simulink subsystem "PvtSubSys_LSM"  (R2020b)
settings: Solver=VariableStepAuto  StartTime=0.0  StopTime=10.0  RelTol=1e-3
values from neighbouring files (symbols this model uses):
  P_LSM_ALC_Enable = 0.0    [LSM_Parameter.sldd]
  P_LSM_DOP_C0_EN_Limit = 0.8    [LSM_Parameter.sldd]
  P_LSM_DOP_C0_out_Limit = 2.0    [LSM_Parameter.sldd]
  P_LSM_DOP_C1_EN_Limit : value not decoded    [LSM_Parameter.sldd]
  P_LSM_DOP_C1_out_Limit : value not decoded    [LSM_Parameter.sldd]
  P_LSM_DOP_C1AndC2_Lim_X : value not decoded    [LSM_Parameter.sldd]
  P_LSM_DOP_C2_EN_Limit : value not decoded    [LSM_Parameter.sldd]
  P_LSM_DOP_C2_out_Limit : value not decoded    [LSM_Parameter.sldd]
  P_LSM_DOP_In_Pre2Dop_Dis = 1.0    [LSM_Parameter.sldd]
  P_LSM_DOP_Out_Pre2Dop_Dis = 2.0    [LSM_Parameter.sldd]
  P_LSM_DOP_PreDis_X : value not decoded    [LSM_Parameter.sldd]
  P_LSM_DOP_PreDis_Y : value not decoded    [LSM_Parameter.sldd]
  P_LSM_DOPValid_CheckTime = 0.06    [LSM_Parameter.sldd]
  P_LSM_DoubleLine_Curr2Cent_Dislimit = 0.5    [LSM_Parameter.sldd]
  P_LSM_DoubleLine_Dop2Cent_Dislimit = 0.5    [LSM_Parameter.sldd]
  P_LSM_DoubleLine_DOPOut_C1 : value not decoded    [LSM_Parameter.sldd]
  P_LSM_DoubleLine_Pre2Cent_Dislimit = 1.0    [LSM_Parameter.sldd]
  P_LSM_IFV2CenterAxis = 0.0    [LSM_Parameter.sldd]
  P_LSM_IFV2RearAxis = 0.0    [LSM_Parameter.sldd]
  P_LSM_LineSTD_Limit = 0.15    [LSM_Parameter.sldd]
  P_LSM_NOH_Switch = 0.0    [LSM_Parameter.sldd]
  P_LSM_Pre_t = 0.0    [LSM_Parameter.sldd]
  P_LSM_SingleLine_Cent2Edge_Dislimit = 100.0    [LSM_Parameter.sldd]
  P_LSM_SingleLine_Curr2Cent_Dislimit = 0.2    [LSM_Parameter.sldd]
  P_LSM_SingleLine_Dop2Cent_Dislimit = 0.2    [LSM_Parameter.sldd]
  P_LSM_SingleLine_DOPOut_C1 : value not decoded    [LSM_Parameter.sldd]
  P_LSM_SingleLine_Pre2Cent_Dislimit = 0.5    [LSM_Parameter.sldd]
undefined symbols (not defined in the file or in its folder): P_LSM_LineWijCal_C12, P_LSM_LineWijCal_C13, P_LSM_PosLineLcFac
libraries: simulink x92, TrueDurationTime x2
(part 6 of 9)

== matlab function PvtSubSys_LSM/Subsystem/TargetLineCalc_20ms/Simulink Function/MATLAB Function3 ==
  data: IFV2RearAxis input single size=1; a0 output single size=1; a1 output single size=1; a2 output single size=1; a3 output single size=1; IFV2CenterAxis input single size=1; A0 input single size=1; A1 input single size=1; A2 input single size=1; A3 input single size=1; Range_min input single size=1; Rmin output single size=1; Range_max input single size=1; Rmax output single size=1
function [a0,a1,a2,a3,Rmin,Rmax] = ...
    fcn(IFV2RearAxis,IFV2CenterAxis,A0,A1,A2,A3,Range_min,Range_max)

Rmin = Range_min + IFV2RearAxis;
Rmax = Range_max + IFV2RearAxis;

if Range_max>0
   xi = [10;20;40;80];
   yi = -A3*xi.^3 - A2*xi.^2 - A1*xi - A0 + IFV2CenterAxis;
   xi = xi + IFV2RearAxis;
   [a3,a2,a1,a0] = pl(xi,yi);
else
    a3 = single(0);
    a2 = single(0);
    a1 = single(0);
    a0 = single(0);
end

== matlab function PvtSubSys_LSM/Subsystem/TargetLineCalc_20ms/TargetLineCalc/CalcEgoVehMove ==
  data: dDeltaX output single size=1; tCycle input single size=1; Kap input single size=1; Vego input single size=1; dDeltaY output single size=1; CosOfPsi output single size=1; SinOfPsi output single size=1
function [dDeltaX,dDeltaY,CosOfPsi,SinOfPsi] = EgoVehicleMovement(tCycle,Kap,Vego)
%#codegen
if Kap==0
    dDeltaX = Vego*tCycle;
    dDeltaY = single(0);
    CosOfPsi = single(1);
    SinOfPsi = single(0);
else
    t_Psi = Kap*Vego*tCycle;
    SinOfPsi = sin(t_Psi);
    CosOfPsi = cos(t_Psi);
    dDeltaX = SinOfPsi/Kap;
    dDeltaY = 2*(sin(t_Psi/2)*sin(t_Psi/2))/Kap;
end

== matlab function PvtSubSys_LSM/Subsystem/TargetLineCalc_20ms/TargetLineCalc/VisLineFilter3 ==
  data: DoubleLineLost_b output; LeftOffset_b output boolean; RightOffset_b output boolean; Quality output single; tCycle input single size=1; vRef input; CentLineValid input boolean size=1; CentLineA3 input single size=1; CentLineA2 input single size=1; CentLineA1 input single size=1; CentLineA0 input single; CentLineRange input single; CentQ input single size=1; RoadWidth input; LineUpdate input boolean size=1; dDeltaX input single size=1; dDeltaY input single size=1; CosOfPsi input single size=1; SinOfPsi input single size=1; QualityK1 input single; LineValidK1 input boolean size=1; A3K1 input single size=1; A2K1 input single size=1; A1K1 input single size=1; A0K1 input single size=1; RangeK1 input single size=1; tLostK1 input single size=1; LineValid output boolean size=1; A3 output single size=1; A2 output single size=1; A1 output single size=1; A0 output single size=1; Range output single size=1; tLost output single size=1
function [DoubleLineLost_b,LeftOffset_b,RightOffset_b,Quality,LineValid,A3,A2,A1,A0,Range,tLost] = ...
    VisFilter(tCycle,vRef,CentLineValid,CentLineA3,CentLineA2,CentLineA1,CentLineA0,CentLineRange, CentQ, RoadWidth,LineUpdate,...
    dDeltaX,dDeltaY,CosOfPsi,SinOfPsi,...
    QualityK1,LineValidK1,A3K1,A2K1,A1K1,A0K1,RangeK1,tLostK1)

if (CentLineValid==true)&&(LineUpdate==true)
    LineValid = true;
    A3 = CentLineA3;
    A2 = CentLineA2;
    A1 = CentLineA1;
    A0 = CentLineA0;
    Range = CentLineRange;
    Quality=single(CentQ);
    %     if Range<RangeK1
    %         Range = RangeK1 - vRef*tCycle;
    %     end
    tLost = single(0);
else
    tLost = min(tLostK1 + tCycle,single(10));
    if (LineValidK1==true)&&(tLost<0.5)
        xi = [0;0.25*RangeK1;0.5*RangeK1;RangeK1];
        yi = A3K1*xi.^3 + A2K1*xi.^2 + A1K1*xi + A0K1;
        t_dx = xi-dDeltaX;
        t_dy = yi-dDeltaY;
        TmpX = t_dx*CosOfPsi+t_dy*SinOfPsi;
        TmpY = -t_dx*SinOfPsi+t_dy*CosOfPsi;
        [A3,A2,A1,A0] = pl(TmpX,TmpY);
        LineValid = true;
        Quality=QualityK1;
        Range = RangeK1;
        if Range<5
            LineValid = false;
        end
    else
        LineValid = false;
        A3 = single(0);
        A2 = single(0);
        A1 = single(0);
        A0 = single(0);
        Range = single(0);
        Quality=single(0);
    end
end

if (A0>0)&&(A0K1<0)&&...
        (abs(A0-A0K1)>(RoadWidth - single(1.5)))&&...
        (LineValid==true)&&(LineValidK1==true)
    LeftOffset_b = true;
else
    LeftOffset_b = false;
end
if (A0<0)&&(A0K1>0)&&...
        (abs(A0-A0K1)>(RoadWidth - single(1.5)))&&...
        (LineValid==true)&&(LineValidK1==true)
    RightOffset_b = true;
else
    RightOffset_b = false;
end


if LineValid==false
    DoubleLineLost_b = true;
else
    DoubleLineLost_b = false;
end

== matlab function PvtSubSys_LSM/Subsystem/TargetLineCalc_20ms/TargetLineCalc/CalcEgoVehMove2 ==
  data: dDeltaX output single size=1; tCycle input single size=1; Kap input single size=1; Vego input single size=1; dDeltaY output single size=1; CosOfPsi output single size=1; SinOfPsi output single size=1
function [dDeltaX,dDeltaY,CosOfPsi,SinOfPsi] = EgoVehicleMovement(tCycle,Kap,Vego)
%#codegen
if Kap==0
    dDeltaX = Vego*tCycle;
    dDeltaY = single(0);
    CosOfPsi = single(1);
    SinOfPsi = single(0);
else
    t_Psi = Kap*Vego*tCycle;
    SinOfPsi = sin(t_Psi);
    CosOfPsi = cos(t_Psi);
    dDeltaX = SinOfPsi/Kap;
    dDeltaY = 2*(sin(t_Psi/2)*sin(t_Psi/2))/Kap;
end

== matlab function PvtSubSys_LSM/Subsystem/TargetLineCalc_20ms/TargetLineCalc/ESSLineCalc ==
  data: LeftLineTypeEn input boolean size=1; ESSLineValid output boolean size=1; RightLineTypeEn input boolean size=1; ESSSts input uint8 size=1; ESSStsK1 input uint8 size=1; LineConf input uint8 size=4; A3 input single size=4; A2 input single size=4; A1 input single size=4; A0 input single size=4; Range input single size=4; tLost input single size=4; EdgeValid input boolean size=2; EdgeA3 input single size=2; EdgeA2 input single size=2; EdgeA1 input single size=2; EdgeA0 input single size=2; dDeltaX input single size=1; dDeltaY input single size=1; CosOfPsi input single size=1; SinOfPsi input single size=1; LeftOffset_b input boolean size=1; RightOffset_b input boolean size=1; RoadWidth input single size=1; ESSDistLim input single size=1; ESSLineA3K1 input single size=1; ESSLineA2K1 input single size=1; ESSLineA1K1 input single size=1; ESSLineA0K1 input single size=1; ESSLeLineA3K1 input single size=1; ESSLineLA2K1 input single size=1; ESSLineLA1K1 input single size=1; ESSLineLA0K1 input single size=1; ESSLineRA3K1 input single size=1; ESSLineRA2K1 input single size=1; ESSLineRA1K1 input single size=1; ESSLineRA0K1 input single size=1; MoveIDK1 input int8 size=1; ESSLineC3 output single size=1; ESSLineC2 output single size=1; ESSLineC1 output single size=1; ESSLineC0 output single size=1; ESSRange output single size=1; ESSLeLineValid output boolean size=1; ESSLeLineC3 output single size=1; ESSLeLineC2 output single size=1; ESSLeLineC1 output single size=1; ESSLeLineC0 output single size=1; ESSLeRange output single size=1; ESSRiLineValid output boolean size=1; ESSRiLineC3 output single size=1; ESSRiLineC2 output single size=1; ESSRiLineC1 output single size=1; ESSRiLineC0 output single size=1; ESSRiRange output single size=1; MoveID output int8 size=1; Lock_bK1 input boolean size=1; Lock_b output boolean size=1
function [ESSLineValid,ESSLineC3,ESSLineC2,ESSLineC1,ESSLineC0,ESSRange,...
    ESSLeLineValid,ESSLeLineC3,ESSLeLineC2,ESSLeLineC1,ESSLeLineC0,ESSLeRange,...
    ESSRiLineValid,ESSRiLineC3,ESSRiLineC2,ESSRiLineC1,ESSRiLineC0,ESSRiRange,MoveID,Lock_b] = ...
    LineCalc(LeftLineTypeEn,RightLineTypeEn,ESSSts,ESSStsK1,LineConf,A3,A2,A1,A0,Range,tLost,...
    EdgeValid,EdgeA3,EdgeA2,EdgeA1,EdgeA0,...
    dDeltaX,dDeltaY,CosOfPsi,SinOfPsi,...
    LeftOffset_b,RightOffset_b,RoadWidth,ESSDistLim,...
    ESSLineA3K1,ESSLineA2K1,ESSLineA1K1,ESSLineA0K1,...
    ESSLeLineA3K1,ESSLineLA2K1,ESSLineLA1K1,ESSLineLA0K1,...
    ESSLineRA3K1,ESSLineRA2K1,ESSLineRA1K1,ESSLineRA0K1,...
    MoveIDK1,Lock_bK1)

ESSLineValid = false;
ESSLineC3 = single(0);
ESSLineC2 = single(0);
ESSLineC1 = single(0);
ESSLineC0 = single(0);
ESSRange = single(0);
ESSLeLineValid = false;
ESSLeLineC3 = single(0);
ESSLeLineC2 = single(0);
ESSLeLineC1 = single(0);
ESSLeLineC0 = single(0);
ESSLeRange = single(0);
ESSRiLineValid = false;
ESSRiLineC3 = single(0);
ESSRiLineC2 = single(0);
ESSRiLineC1 = single(0);
ESSRiLineC0 = single(0);
ESSRiRange = single(0);

MoveID = MoveIDK1;
Lock_b = Lock_bK1;

if (ESSSts==0)||(ESSSts==1)||(ESSSts==2)||(ESSSts==6)
    MoveID = int8(0);
    Lock_b = false;
%     if (LineConf(2)>0)&&(LineConf(3)>0)&&...
%             (Range(2)>ESSDistLim)&&(Range(3)>ESSDistLim)&&...
%             ((tLost(2)<0.15)||(tLost(3)<0.15))
%             ESSLineValid = true;
%             ESSLineA3 = 0.5*(A3(2) + A3(3));
%             ESSLineA2 = 0.5*(A2(2) + A2(3));
%             ESSLineA1 = 0.5*(A1(2) + A1(3));
%             ESSLineA0 = 0.5*(A0(2) + A0(3));
%             ESSLineRange = 0.5*(Range(2) + Range(3));
%     end
    if (LineConf(2)>0)&&(LineConf(1)>0)&&...
            (Range(2)>ESSDistLim)&&(Range(1)>ESSDistLim)&&...
            ((tLost(2)<0.15)||(tLost(1)<0.15))&&...
            (LeftLineTypeEn) && abs(A0(1)-A0(2))>3
        
        if EdgeValid(1)==true
            t = [0.1*ESSDistLim;0.3*ESSDistLim;0.6*ESSDistLim;ESSDistLim];
            t_EdgeDy = 0.25*EdgeA3(1)*t.^3 + 0.5*EdgeA2(1)*t.^2 + EdgeA1(1)*t + EdgeA0(1);
            t_LineLDy = A3(1)*t.^3 + A2(1)*t.^2 + A1(1)*t + A0(1);
            if min(t_EdgeDy - t_LineLDy)>0
                ESSLeLineValid = true;
                ESSLeLineC3 = 0.5*(A3(2) + A3(1));
                ESSLeLineC2 = 0.5*(A2(2) + A2(1));
                ESSLeLineC1 = 0.5*(A1(2) + A1(1));
                ESSLeLineC0 = 0.5*(A0(2) + A0(1));
                ESSLeRange = 0.5*(Range(2) + Range(1));
            end
        else
            ESSLeLineValid = true;
            ESSLeLineC3 = 0.5*(A3(2) + A3(1));
            ESSLeLineC2 = 0.5*(A2(2) + A2(1));
            ESSLeLineC1 = 0.5*(A1(2) + A1(1));
            ESSLeLineC0 = 0.5*(A0(2) + A0(1));
            ESSLeRange = 0.5*(Range(2) + Range(1));
        end
    end
    if (LineConf(4)>0)&&(LineConf(3)>0)&&...
            (Range(4)>ESSDistLim)&&(Range(3)>ESSDistLim)&&...
            ((tLost(4)<0.15)||(tLost(3)<0.15))&&...
            (RightLineTypeEn) && abs(A0(3)-A0(4))>3
        
        if EdgeValid(2)==true
            t = [0.1*ESSDistLim;0.3*ESSDistLim;0.6*ESSDistLim;ESSDistLim];
            t_EdgeDy = 0.25*EdgeA3(2)*t.^3 + 0.5*EdgeA2(2)*t.^2 + EdgeA1(2)*t + EdgeA0(2);
            t_LineLDy = A3(4)*t.^3 + A2(4)*t.^2 + A1(4)*t + A0(4);
            if min(t_LineLDy - t_EdgeDy)>0
                ESSRiLineValid = true;
                ESSRiLineC3 = 0.5*(A3(4) + A3(3));
                ESSRiLineC2 = 0.5*(A2(4) + A2(3));
                ESSRiLineC1 = 0.5*(A1(4) + A1(3));
                ESSRiLineC0 = 0.5*(A0(4) + A0(3));
                ESSRiRange = 0.5*(Range(4) + Range(3));
            end
        else
            ESSRiLineValid = true;
            ESSRiLineC3 = 0.5*(A3(4) + A3(3));
            ESSRiLineC2 = 0.5*(A2(4) + A2(3));
            ESSRiLineC1 = 0.5*(A1(4) + A1(3));
            ESSRiLineC0 = 0.5*(A0(4) + A0(3));
            ESSRiRange = 0.5*(Range(4) + Range(3));
        end
    end
elseif ESSSts==4
    if ESSStsK1~=4
        MoveID = MoveID - int8(1);
    end
    if LeftOffset_b
        MoveID = MoveID + int8(1);
    end
    if RightOffset_b
        MoveID = MoveID - int8(1);
    end
    if (MoveID>=1)||(MoveID<=-2)
        Error = true;
    else
        Error = false;
    end
    if Error==false
        if (LineConf(int8(2)+MoveID)>0)&&(LineConf(int8(3)+MoveID)>0)&&...
                (Range(int8(2)+MoveID)>0.8*ESSDistLim)&&(Range(int8(3)+MoveID)>0.8*ESSDistLim)
            Lock_b = false;
            ESSLineValid = true;
            ESSLineC3 = 0.5*(A3(int8(2)+MoveID) + A3(int8(3)+MoveID));
            ESSLineC2 = 0.5*(A2(int8(2)+MoveID) + A2(int8(3)+MoveID));
            ESSLineC1 = 0.5*(A1(int8(2)+MoveID) + A1(int8(3)+MoveID));
            ESSLineC0 = 0.5*(A0(int8(2)+MoveID) + A0(int8(3)+MoveID));
            ESSRange = 0.5*(Range(int8(2)+MoveID) + Range(int8(3)+MoveID));
            
            ESSLeLineValid = true;
            ESSLeLineC3 = 0.5*(A3(int8(2)+MoveID) + A3(int8(3)+MoveID));
            ESSLeLineC2 = 0.5*(A2(int8(2)+MoveID) + A2(int8(3)+MoveID));
            ESSLeLineC1 = 0.5*(A1(int8(2)+MoveID) + A1(int8(3)+MoveID));
            ESSLeLineC0 = 0.5*(A0(int8(2)+MoveID) + A0(int8(3)+MoveID));
            ESSLeRange = 0.5*(Range(int8(2)+MoveID) + Range(int8(3)+MoveID));
           elseif (LineConf(int8(2)+MoveID)>0)&&(Range(int8(2)+MoveID)>0.8*ESSDistLim)
            Lock_b = true;
            ESSLineValid = true;
            ESSLineA3 = A3(2+MoveID);
            ESSLineA2 = A2(2+MoveID);
            ESSLineA1 = A1(2+MoveID);
            ESSLineA0 = A0(2+MoveID)-0.5*RoadWidth*sqrt(1+A1(2+MoveID)*A1(2+MoveID));
            ESSLineRange = Range(2+MoveID);
            ESSLeLineValid = true;
            ESSLeLineA3 = ESSLineA3;
            ESSLeLineA2 = ESSLineA2;
            ESSLeLineA1 = ESSLineA1;
            ESSLeLineA0 = ESSLineA0;
            ESSLeRange =ESSLineRange;
%             SingleLineLost_b = true;
        elseif (LineConf(int8(3)+MoveID)>0)&&(Range(int8(3)+MoveID)>0.8*ESSDistLim)
            Lock_b = true;
            ESSLineValid = true;
            ESSLineA3 = A3(3+MoveID);
            ESSLineA2 = A2(3+MoveID);
            ESSLineA1 = A1(3+MoveID);
            ESSLineA0 = A0(3+MoveID)+0.5*RoadWidth*sqrt(1+A1(3+MoveID)*A1(3+MoveID));
            ESSLineRange = Range(3+MoveID);
            ESSLeLineValid = true;
            ESSLeLineA3 = ESSLineA3;
            ESSLeLineA2 = ESSLineA2;
            ESSLeLineA1 = ESSLineA1;
            ESSLeLineA0 = ESSLineA0;
            ESSLeRange =ESSLineRange;
%             SingleLineLost_b = true; 
%         else
%             Lock_b = true;
%             MoveID = int8(0);
%             if ESSStsK1~=4
%                 xi = [0;10;20;40];
%                 yi = ESSLineLA3K1*xi.^3 + ESSLineLA2K1*xi.^2 + ESSLineLA1K1*xi + ESSLineLA0K1;
%                 t_dx = xi-dDeltaX;
%                 t_dy = yi-dDeltaY;
%                 TmpX = t_dx*CosOfPsi+t_dy*SinOfPsi;
%                 TmpY = -t_dx*SinOfPsi+t_dy*CosOfPsi;
%                 [ESSLineC3,ESSLineC2,ESSLineC1,ESSLineC0] = pl(TmpX,TmpY);
%                 ESSLineValid = true;
%             else
%                 xi = [0;10;20;40];
%                 yi = ESSLineA3K1*xi.^3 + ESSLineA2K1*xi.^2 + ESSLineA1K1*xi + ESSLineA0K1;
%                 t_dx = xi-dDeltaX;
%                 t_dy = yi-dDeltaY;
%                 TmpX = t_dx*CosOfPsi+t_dy*SinOfPsi;
%                 TmpY = -t_dx*SinOfPsi+t_dy*CosOfPsi;
%                 [ESSLineC3,ESSLineC2,ESSLineC1,ESSLineC0] = pl(TmpX,TmpY);
%                 ESSLineValid = true;
            end
        end
    end
elseif ESSSts==5
    if ESSStsK1~=5
        MoveID = MoveID + int8(1);
    end
    if LeftOffset_b
        MoveID = MoveID + int8(1);
    end
    if RightOffset_b
        MoveID = MoveID - int8(1);
    end
    if (MoveID>=2)||(MoveID<=-1)
        Error = true;
    else
        Error = false;
    end
    if Error==false
        if (Lock_b==false)&&...
                (LineConf(int8(2)+MoveID)>0)&&(LineConf(int8(3)+MoveID)>0)&&...
                (Range(int8(2)+MoveID)>0.8*ESSDistLim)&&(Range(int8(3)+MoveID)>0.8*ESSDistLim)
            
            ESSLineValid = true;
            ESSLineC3 = 0.5*(A3(int8(2)+MoveID) + A3(int8(3)+MoveID));
            ESSLineC2 = 0.5*(A2(int8(2)+MoveID) + A2(int8(3)+MoveID));
            ESSLineC1 = 0.5*(A1(int8(2)+MoveID) + A1(int8(3)+MoveID));
            ESSLineC0 = 0.5*(A0(int8(2)+MoveID) + A0(int8(3)+MoveID));
            ESSRange = 0.5*(Range(int8(2)+MoveID) + Range(int8(3)+MoveID));
            
            ESSRiLineValid = true;
            ESSRiLineC3 = 0.5*(A3(int8(2)+MoveID) + A3(int8(3)+MoveID));
            ESSRiLineC2 = 0.5*(A2(int8(2)+MoveID) + A2(int8(3)+MoveID));
            ESSRiLineC1 = 0.5*(A1(int8(2)+MoveID) + A1(int8(3)+MoveID));
            ESSRiLineC0 = 0.5*(A0(int8(2)+MoveID) + A0(int8(3)+MoveID));
            ESSRiRange = 0.5*(Range(int8(2)+MoveID) + Range(int8(3)+MoveID));
        else
            Lock_b = true;
            MoveID = int8(0);
            if ESSStsK1~=5
                xi = [0;10;20;40];
                yi = ESSLineRA3K1*xi.^3 + ESSLineRA2K1*xi.^2 + ESSLineRA1K1*xi + ESSLineRA0K1;
                t_dx = xi-dDeltaX;
                t_dy = yi-dDeltaY;
                TmpX = t_dx*CosOfPsi+t_dy*SinOfPsi;
                TmpY = -t_dx*SinOfPsi+t_dy*CosOfPsi;
                [ESSLineC3,ESSLineC2,ESSLineC1,ESSLineC0] = pl(TmpX,TmpY);
                ESSLineValid = true;
            else
                xi = [0;10;20;40];
                yi = ESSLineA3K1*xi.^3 + ESSLineA2K1*xi.^2 + ESSLineA1K1*xi + ESSLineA0K1;
                t_dx = xi-dDeltaX;
                t_dy = yi-dDeltaY;
                TmpX = t_dx*CosOfPsi+t_dy*SinOfPsi;
                TmpY = -t_dx*SinOfPsi+t_dy*CosOfPsi;
                [ESSLineC3,ESSLineC2,ESSLineC1,ESSLineC0] = pl(TmpX,TmpY);
                ESSLineValid = true;
            end
        end
    end 
end
end

== matlab function PvtSubSys_LSM/Subsystem/TargetLineCalc_20ms/TargetLineCalc/ESSLineCalc1 ==
  data: LeftLineTypeEn input boolean; ESSLineValid output boolean; RightLineTypeEn input boolean; ESSSts input uint8; ESSStsK1 input uint8; LineConf input uint8; A3 input single; A2 input single; A1 input single; A0 input single; Range input single; tLost input single; EdgeValid input boolean; EdgeA3 input single; EdgeA2 input single; EdgeA1 input single; EdgeA0 input single; LeftOffset_b input boolean; RightOffset_b input boolean; RoadWidth input single; ESSDistLim input single; MoveIDK1 input int8; ESSLineA3 output single; ESSLineA2 output single; ESSLineA1 output single; ESSLineA0 output single; ESSRange output single; ESSLeLineValid output boolean; ESSLeLineA3 output single; ESSLeLineA2 output single; ESSLeLineA1 output single; ESSLeLineA0 output single; ESSLeRange output single; ESSRiLineValid output boolean; ESSRiLineA3 output single; ESSRiLineA2 output single; ESSRiLineA1 output single; ESSRiLineA0 output single; ESSRiRange output single; MoveID output int8; Lock_bK1 input boolean; Lock_b output boolean
function [ESSLineValid,ESSLineA3,ESSLineA2,ESSLineA1,ESSLineA0,ESSRange,...
    ESSLeLineValid,ESSLeLineA3,ESSLeLineA2,ESSLeLineA1,ESSLeLineA0,ESSLeRange,...
    ESSRiLineValid,ESSRiLineA3,ESSRiLineA2,ESSRiLineA1,ESSRiLineA0,ESSRiRange,MoveID,Lock_b] = ...
    LineCalc(LeftLineTypeEn,RightLineTypeEn,ESSSts,ESSStsK1,LineConf,A3,A2,A1,A0,Range,tLost,...
    EdgeValid,EdgeA3,EdgeA2,EdgeA1,EdgeA0,...
    LeftOffset_b,RightOffset_b,RoadWidth,ESSDistLim,...
    MoveIDK1,Lock_bK1)

ESSLineValid = false;
ESSLineA3 = single(0);
ESSLineA2 = single(0);
ESSLineA1 = single(0);
ESSLineA0 = single(0);
ESSRange = single(0);
ESSLeLineValid = false;
ESSLeLineA3 = single(0);
ESSLeLineA2 = single(0);
ESSLeLineA1 = single(0);
ESSLeLineA0 = single(0);
ESSLeRange = single(0);
ESSRiLineValid = false;
ESSRiLineA3 = single(0);
ESSRiLineA2 = single(0);
ESSRiLineA1 = single(0);
ESSRiLineA0 = single(0);
ESSRiRange = single(0);
% SingleLineLost_b = false;
% DoubleLineLost_b = false;
MoveID = MoveIDK1;
Lock_b = Lock_bK1;

if (ESSSts==0)||(ESSSts==1)||(ESSSts==2)||(ESSSts==6)
    MoveID = int8(0);
    Lock_b = false;             %add
%         if (LineConf(2)>0)&&(LineConf(3)>0)&&...
%                 (Range(2)>ESSDistLim)&&(Range(3)>ESSDistLim)&&...
%                 ((tLost(2)<0.15)||(tLost(3)<0.15))
%                 ESSLineValid = true;
%                 ESSLineA3 = 0.5*(A3(2) + A3(3));
%                 ESSLineA2 = 0.5*(A2(2) + A2(3));
%                 ESSLineA1 = 0.5*(A1(2) + A1(3));
%                 ESSLineA0 = 0.5*(A0(2) + A0(3));
%                 ESSLineRange = 0.5*(Range(2) + Range(3));
%         end
    if (LineConf(2)>0)&&(LineConf(1)>0)&&...
            (Range(2)>ESSDistLim)&&(Range(1)>ESSDistLim)&&...
            ((tLost(2)<0.15)||(tLost(1)<0.15))&&...
            (LeftLineTypeEn)
        
        if EdgeValid(1)==true
            t = [0.1*ESSDistLim;0.3*ESSDistLim;0.6*ESSDistLim;ESSDistLim];
            t_EdgeDy = 0.25*EdgeA3(1)*t.^3 + 0.5*EdgeA2(1)*t.^2 + EdgeA1(1)*t + EdgeA0(1);
            t_LineLDy = A3(1)*t.^3 + A2(1)*t.^2 + A1(1)*t + A0(1);
            if min(t_EdgeDy - t_LineLDy)>0
                ESSLeLineValid = true;
                ESSLeLineA3 = 0.5*(A3(2) + A3(1));
                ESSLeLineA2 = 0.5*(A2(2) + A2(1));
                ESSLeLineA1 = 0.5*(A1(2) + A1(1));
                ESSLeLineA0 = 0.5*(A0(2) + A0(1));
                ESSLeRange = 0.5*(Range(2) + Range(1));
            end
        else
            ESSLeLineValid = true;
            ESSLeLineA3 = 0.5*(A3(2) + A3(1));
            ESSLeLineA2 = 0.5*(A2(2) + A2(1));
            ESSLeLineA1 = 0.5*(A1(2) + A1(1));
            ESSLeLineA0 = 0.5*(A0(2) + A0(1));
            ESSLeRange = 0.5*(Range(2) + Range(1));
        end
    end
    if (LineConf(4)>0)&&(LineConf(3)>0)&&...
            (Range(4)>ESSDistLim)&&(Range(3)>ESSDistLim)&&...
            ((tLost(4)<0.15)||(tLost(3)<0.15))&&...
            (RightLineTypeEn)
        
        if EdgeValid(2)==true
            t = [0.1*ESSDistLim;0.3*ESSDistLim;0.6*ESSDistLim;ESSDistLim];
            t_EdgeDy = 0.25*EdgeA3(2)*t.^3 + 0.5*EdgeA2(2)*t.^2 + EdgeA1(2)*t + EdgeA0(2);
            t_LineLDy = A3(4)*t.^3 + A2(4)*t.^2 + A1(4)*t + A0(4);
            if min(t_LineLDy - t_EdgeDy)>0
                ESSRiLineValid = true;
                ESSRiLineA3 = 0.5*(A3(4) + A3(3));
                ESSRiLineA2 = 0.5*(A2(4) + A2(3));
                ESSRiLineA1 = 0.5*(A1(4) + A1(3));
                ESSRiLineA0 = 0.5*(A0(4) + A0(3));
                ESSRiRange = 0.5*(Range(4) + Range(3));
            end
        else
            ESSRiLineValid = true;
            ESSRiLineA3 = 0.5*(A3(4) + A3(3));
            ESSRiLineA2 = 0.5*(A2(4) + A2(3));
            ESSRiLineA1 = 0.5*(A1(4) + A1(3));
            ESSRiLineA0 = 0.5*(A0(4) + A0(3));
            ESSRiRange = 0.5*(Range(4) + Range(3));
        end
    end
elseif ESSSts==4
    if ESSStsK1~=4
        MoveID = MoveID - int8(1);
    end
    if LeftOffset_b
        MoveID = MoveID + int8(1);
    end
    if RightOffset_b
        MoveID = MoveID - int8(1);
    end
    if (MoveID>=1)||(MoveID<=-2)
        Error = true;
    else
        Error = false;
    end
    if Error==false
        if  (LineConf(int8(2)+MoveID)>0)&&(LineConf(int8(3)+MoveID)>0)&&...
                (Range(int8(2)+MoveID)>0.8*ESSDistLim)&&(Range(int8(3)+MoveID)>0.8*ESSDistLim)
%                 &&(abs(A0(int8(2)+MoveID)-A0(int8(3)+MoveID))>=0.8*RoadWidth)...     %add
%                 &&(VisLineConf(int8(2)+MoveID)>0)&&(VisLineConf(int8(3)+MoveID)>0)   %add
            Lock_b = false;
            ESSLineValid = true;
            ESSLineA3 = 0.5*(A3(int8(2)+MoveID) + A3(int8(3)+MoveID));
            ESSLineA2 = 0.5*(A2(int8(2)+MoveID) + A2(int8(3)+MoveID));
            ESSLineA1 = 0.5*(A1(int8(2)+MoveID) + A1(int8(3)+MoveID));
            ESSLineA0 = 0.5*(A0(int8(2)+MoveID) + A0(int8(3)+MoveID));
            ESSRange = 0.5*(Range(int8(2)+MoveID) + Range(int8(3)+MoveID));
            
            ESSLeLineValid = true;
            ESSLeLineA3 = 0.5*(A3(int8(2)+MoveID) + A3(int8(3)+MoveID));
            ESSLeLineA2 = 0.5*(A2(int8(2)+MoveID) + A2(int8(3)+MoveID));
            ESSLeLineA1 = 0.5*(A1(int8(2)+MoveID) + A1(int8(3)+MoveID));
            ESSLeLineA0 = 0.5*(A0(int8(2)+MoveID) + A0(int8(3)+MoveID));
            ESSLeRange = 0.5*(Range(int8(2)+MoveID) + Range(int8(3)+MoveID));
        elseif (LineConf(int8(2)+MoveID)>0)&&(Range(int8(2)+MoveID)>0.8*ESSDistLim)
            Lock_b = true;
            ESSLineValid = true;
            ESSLineA3 = A3(2+MoveID);
            ESSLineA2 = A2(2+MoveID);
            ESSLineA1 = A1(2+MoveID);
            ESSLineA0 = A0(2+MoveID)-0.5*RoadWidth*sqrt(1+A1(2+MoveID)*A1(2+MoveID));
            ESSRange = Range(2+MoveID);
            ESSLeLineValid = true;
            ESSLeLineA3 = ESSLineA3;
            ESSLeLineA2 = ESSLineA2;
            ESSLeLineA1 = ESSLineA1;
            ESSLeLineA0 = ESSLineA0;
            ESSLeRange =ESSRange;
        elseif (LineConf(int8(3)+MoveID)>0)&&(Range(int8(3)+MoveID)>0.8*ESSDistLim)
            Lock_b = true;
            ESSLineValid = true;
            ESSLineA3 = A3(3+MoveID);
            ESSLineA2 = A2(3+MoveID);
            ESSLineA1 = A1(3+MoveID);
            ESSLineA0 = A0(3+MoveID)+0.5*RoadWidth*sqrt(1+A1(3+MoveID)*A1(3+MoveID));
            ESSRange = Range(3+MoveID);
            ESSLeLineValid = true;
            ESSLeLineA3 = ESSLineA3;
            ESSLeLineA2 = ESSLineA2;
            ESSLeLineA1 = ESSLineA1;
            ESSLeLineA0 = ESSLineA0;
            ESSLeRange =ESSRange;
            %             MoveID = int8(0);
%             if ESSStsK1~=4
%                 xi = [0;10;20;40];
%                 yi = ESSLineLA3K1*xi.^3 + ESSLineLA2K1*xi.^2 + ESSLineLA1K1*xi + ESSLineLA0K1;
%                 t_dx = xi-dDeltaX;
%                 t_dy = yi-dDeltaY;
%                 TmpX = t_dx*CosOfPsi+t_dy*SinOfPsi;
%                 TmpY = -t_dx*SinOfPsi+t_dy*CosOfPsi;
%                 [ESSLineLA3,ESSLineLA2,ESSLineLA1,ESSLineLA0] = pl(TmpX,TmpY);
%                 ESSLineLValid = true;
%                 [ESSLineA3,ESSLineA2,ESSLineA1,ESSLineA0] = pl(TmpX,TmpY);
%                 ESSLineValid = true;
%             else
%                 xi = [0;10;20;40];
%                 yi = ESSLineLA3K1*xi.^3 + ESSLineLA2K1*xi.^2 + ESSLineLA1K1*xi + ESSLineLA0K1;
%                 t_dx = xi-dDeltaX;
%                 t_dy = yi-dDeltaY;
%                 TmpX = t_dx*CosOfPsi+t_dy*SinOfPsi;
%                 TmpY = -t_dx*SinOfPsi+t_dy*CosOfPsi;
%                 [ESSLineLA3,ESSLineLA2,ESSLineLA1,ESSLineLA0] = pl(TmpX,TmpY);
%                 ESSLineLValid = true;
%                 [ESSLineA3,ESSLineA2,ESSLineA1,ESSLineA0] = pl(TmpX,TmpY);
%                 ESSLineValid = true;
%             end
        end
    end
elseif ESSSts==5
    if ESSStsK1~=5
        MoveID = MoveID + int8(1);
    end
    if LeftOffset_b
        MoveID = MoveID + int8(1);
    end
    if RightOffset_b
        MoveID = MoveID - int8(1);
    end
    if (MoveID>=2)||(MoveID<=-1)
        Error = true;
    else
        Error = false;
    end
    if Error==false
        if (LineConf(int8(2)+MoveID)>0)&&(LineConf(int8(3)+MoveID)>0)&&...
                (Range(int8(2)+MoveID)>0.8*ESSDistLim)&&(Range(int8(3)+MoveID)>0.8*ESSDistLim)
%                 &&(abs(A0(int8(2)+MoveID)-A0(int8(3)+MoveID))>=0.8*RoadWidth)...             %add
%                 &&(VisLineConf(int8(2)+MoveID)>0)&&(VisLineConf(int8(3)+MoveID)>0)           %add
            Lock_b = false;
            ESSLineValid = true;
            ESSLineA3 = 0.5*(A3(int8(2)+MoveID) + A3(int8(3)+MoveID));
            ESSLineA2 = 0.5*(A2(int8(2)+MoveID) + A2(int8(3)+MoveID));
            ESSLineA1 = 0.5*(A1(int8(2)+MoveID) + A1(int8(3)+MoveID));
            ESSLineA0 = 0.5*(A0(int8(2)+MoveID) + A0(int8(3)+MoveID));
            ESSRange = 0.5*(Range(int8(2)+MoveID) + Range(int8(3)+MoveID));
            
            ESSRiLineValid = true;
            ESSRiLineA3 = 0.5*(A3(int8(2)+MoveID) + A3(int8(3)+MoveID));
            ESSRiLineA2 = 0.5*(A2(int8(2)+MoveID) + A2(int8(3)+MoveID));
            ESSRiLineA1 = 0.5*(A1(int8(2)+MoveID) + A1(int8(3)+MoveID));
            ESSRiLineA0 = 0.5*(A0(int8(2)+MoveID) + A0(int8(3)+MoveID));
            ESSRiRange = 0.5*(Range(int8(2)+MoveID) + Range(int8(3)+MoveID));
        elseif (LineConf(int8(2)+MoveID)>0)&&(Range(int8(2)+MoveID)>0.8*ESSDistLim)
            Lock_b = true;
            ESSLineValid = true;
            ESSLineA3 = A3(2+MoveID);
            ESSLineA2 = A2(2+MoveID);
            ESSLineA1 = A1(2+MoveID);
            ESSLineA0 = A0(2+MoveID)-0.5*RoadWidth*sqrt(1+A1(2+MoveID)*A1(2+MoveID));
            ESSRange = Range(2+MoveID);
            ESSRiLineValid = true;
            ESSRiLineA3 = ESSLineA3;
            ESSRiLineA2 = ESSLineA2;
            ESSRiLineA1 = ESSLineA1;
            ESSRiLineA0 = ESSLineA0;
            ESSRiRange =ESSRange;
        elseif (LineConf(int8(3)+MoveID)>0)&&(Range(int8(3)+MoveID)>0.8*ESSDistLim)
            Lock_b = true;
            ESSLineValid = true;
            ESSLineA3 = A3(3+MoveID);
            ESSLineA2 = A2(3+MoveID);
            ESSLineA1 = A1(3+MoveID);
            ESSLineA0 = A0(3+MoveID)+0.5*RoadWidth*sqrt(1+A1(3+MoveID)*A1(3+MoveID));
            ESSRange = Range(3+MoveID);
            ESSRiLineValid = true;
            ESSRiLineA3 = ESSLineA3;
            ESSRiLineA2 = ESSLineA2;
            ESSRiLineA1 = ESSLineA1;
            ESSRiLineA0 = ESSLineA0;
            ESSRiRange =ESSRange;
            %             MoveID = int8(0);
%             if ESSStsK1~=5
%                 xi = [0;10;20;40];
%                 yi = ESSLineRA3K1*xi.^3 + ESSLineRA2K1*xi.^2 + ESSLineRA1K1*xi + ESSLineRA0K1;
%                 t_dx = xi-dDeltaX;
%                 t_dy = yi-dDeltaY;
%                 TmpX = t_dx*CosOfPsi+t_dy*SinOfPsi;
%                 TmpY = -t_dx*SinOfPsi+t_dy*CosOfPsi;
%                 [ESSLineA3,ESSLineA2,ESSLineA1,ESSLineA0] = pl(TmpX,TmpY);
%                 ESSLineValid = true;
%                 [ESSLineRA3,ESSLineRA2,ESSLineRA1,ESSLineRA0] = pl(TmpX,TmpY);
%                 ESSLineRValid = true;
%             else
%                 xi = [0;10;20;40];
%                 yi = ESSLineRA3K1*xi.^3 + ESSLineRA2K1*xi.^2 + ESSLineRA1K1*xi + ESSLineRA0K1;
%                 t_dx = xi-dDeltaX;
%                 t_dy = yi-dDeltaY;
%                 TmpX = t_dx*CosOfPsi+t_dy*SinOfPsi;
%                 TmpY = -t_dx*SinOfPsi+t_dy*CosOfPsi;
%                 [ESSLineRA3,ESSLineRA2,ESSLineRA1,ESSLineRA0] = pl(TmpX,TmpY);
%                 ESSLineRValid = true;
%                 [ESSLineA3,ESSLineA2,ESSLineA1,ESSLineA0] = pl(TmpX,TmpY);
%                 ESSLineValid = true;
%             end
        end
    end
end

== matlab function PvtSubSys_LSM/Subsystem/TargetLineCalc_20ms/TargetLineCalc/HWALineCalc ==
  data: HWALineC0K1 input; TJA_Line_State input; HWALineValid output boolean size=1; HWASts input uint8 size=1; HWAStsK1 input uint8 size=1; PathValid input boolean; PathA3 input single; PathA2 input single; PathA1 input single; PathA0 input single; PathRange input; PathLaneAvail input; TJALineValid input; TJALineA3 input; TJALineA2 input; TJALineA1 input; TJALineA0 input; TJALineRange input; LeftOffset_b input boolean size=1; RightOffset_b input boolean size=1; HWALineC3 output single size=1; HWALineC2 output single size=1; HWALineC1 output single size=1; HWALineC0 output single size=1; HWARange output single size=1; dDeltaX input single size=1; dDeltaY input single size=1; CosOfPsi input single size=1; SinOfPsi input single size=1; vRef input single size=1; HWALeLineValid output boolean size=1; HWALeLineC3 output single size=1; HWALeLineC2 output single size=1; HWALeLineC1 output single size=1; HWALeLineC0 output single size=1; HWALeRange output single size=1; HWARiLineValid output boolean size=1; HWARiLineC3 output single size=1; HWARiLineC2 output single size=1; HWARiLineC1 output single size=1; HWARiLineC0 output single size=1; HWARiRange output single size=1; preDyDiff output single size=1; HeadAngDiff output single size=1; Error output boolean size=1; MoveIDK1 input int8 size=1; LockIDK1 input int8; MoveID output int8 size=1; LockID output int8; Lock_counterK1 input uint8; Lock_counter output uint8
function [HWALineValid,HWALineC3,HWALineC2,HWALineC1,HWALineC0,HWARange,...
    HWALeLineValid,HWALeLineC3,HWALeLineC2,HWALeLineC1,HWALeLineC0,HWALeRange,...
    HWARiLineValid,HWARiLineC3,HWARiLineC2,HWARiLineC1,HWARiLineC0,HWARiRange,...
    preDyDiff,HeadAngDiff,Error,MoveID,LockID,Lock_counter] = ...
    LineCalc(HWALineC0K1,TJA_Line_State,HWASts,HWAStsK1,...
    PathValid,PathA3,PathA2,PathA1,PathA0,PathRange,PathLaneAvail,...
    TJALineValid,TJALineA3,TJALineA2,TJALineA1,TJALineA0,TJALineRange,...
    LeftOffset_b,RightOffset_b,dDeltaX,dDeltaY,CosOfPsi,SinOfPsi,vRef,MoveIDK1,LockIDK1,Lock_counterK1)

HWALineValid = false;
HWALineC3 = single(0);
HWALineC2 = single(0);
HWALineC1 = single(0);
HWALineC0 = single(0);
HWARange = single(0);
HWALeLineValid = false;
HWALeLineC3 = single(0);
HWALeLineC2 = single(0);
HWALeLineC1 = single(0);
HWALeLineC0 = single(0);
HWALeRange = single(0);
HWARiLineValid = false;
HWARiLineC3 = single(0);
HWARiLineC2 = single(0);
HWARiLineC1 = single(0);
HWARiLineC0 = single(0);
HWARiRange = single(0);
Error = false;
preDis = single(50);

MoveID = MoveIDK1;
LockID = LockIDK1;
if abs(HWALineC0K1)>4.5
    MoveID = int8(0);
    LockID = int8(0);
end

Lock_counter = max(Lock_counterK1-uint8(1),uint8(0));
if Lock_counter==0
    LockID = int8(0);
end

if (HWASts==1)||(HWASts==7)||(HWASts==0)
    MoveID = int8(0);
end

if HWASts ==1 || HWASts == 2
    HWALineValid = TJALineValid;
    HWALineC3 = TJALineA3;
    HWALineC2 = TJALineA2;
    HWALineC1 = TJALineA1;
    HWALineC0 = TJALineA0;
    HWARange = TJALineRange;
end
if HWASts==3
    MoveID = int8(0);
    if HWAStsK1==5 || HWAStsK1==6
        Lock_counter = uint8(250);
        LockID = int8(0);
    end
    if Lock_counter>0
        if LeftOffset_b
            LockID = LockID + int8(1);
        end
        if RightOffset_b
            LockID = LockID - int8(1);
        end
    end
    
    if LockID==1
        HWALineValid = PathValid(3);
        HWALineC3 = PathA3(3);
        HWALineC2 = PathA2(3);
        HWALineC1 = PathA1(3);
        HWALineC0 = PathA0(3);
        HWARange = PathRange(3);
        
        HWALeLineValid = PathValid(2);
        HWALeLineC3 = PathA3(2);
        HWALeLineC2 = PathA2(2);
        HWALeLineC1 = PathA1(2);
        HWALeLineC0 = PathA0(2);
        HWALeRange = PathRange(2);
        
        HWARiLineValid = PathValid(3);
        HWARiLineC3 = PathA3(3);
        HWARiLineC2 = PathA2(3);
        HWARiLineC1 = PathA1(3);
        HWARiLineC0 = PathA0(3);
        HWARiRange = PathRange(3);
        
    elseif LockID==-1
        HWALineValid = PathValid(1);
        HWALineC3 = PathA3(1);
        HWALineC2 = PathA2(1);
        HWALineC1 = PathA1(1);
        HWALineC0 = PathA0(1);
        HWARange = PathRange(1);
        
        HWALeLineValid = PathValid(1);
        HWALeLineC3 = PathA3(1);
        HWALeLineC2 = PathA2(1);
        HWALeLineC1 = PathA1(1);
        HWALeLineC0 = PathA0(1);
        HWALeRange = PathRange(1);
        
        HWARiLineValid = PathValid(2);
        HWARiLineC3 = PathA3(2);
        HWARiLineC2 = PathA2(2);
        HWARiLineC1 = PathA1(2);
        HWARiLineC0 = PathA0(2);
        HWARiRange = PathRange(2);
    elseif LockID==0
        
        HWALineValid = TJALineValid;
        HWALineC3 = TJALineA3;
        HWALineC2 = TJALineA2;
        HWALineC1 = TJALineA1;
        HWALineC0 = TJALineA0;
        HWARange = TJALineRange;
        
        if PathLaneAvail(1)&&(TJA_Line_State==1)&&(PathA0(1)<4.5)
            HWALeLineValid = PathValid(1);
            HWALeLineC3 = PathA3(1);
            HWALeLineC2 = PathA2(1);
            HWALeLineC1 = PathA1(1);
            HWALeLineC0 = PathA0(1);
            HWALeRange = PathRange(1);
        end
        
        if PathLaneAvail(3)&&(TJA_Line_State==1)&&(PathA0(3)>-4.5)
            HWARiLineValid = PathValid(3);
            HWARiLineC3 = PathA3(3);
            HWARiLineC2 = PathA2(3);
            HWARiLineC1 = PathA1(3);
            HWARiLineC0 = PathA0(3);
            HWARiRange = PathRange(3);
        end
    end
end

if HWASts==5
    if HWAStsK1~=5
        MoveID = MoveID - int8(1);
    end
    if LeftOffset_b
        MoveID = MoveID + int8(1);
    end
    if RightOffset_b
        MoveID = MoveID - int8(1);
    end

    if (MoveID>=1)||(MoveID<=-2)
        Error = true;
    end
    if Error==false
        if MoveID==-1
            HWALineValid = PathValid(1);
            HWALineC3 = PathA3(1);
            HWALineC2 = PathA2(1);
            HWALineC1 = PathA1(1);
            HWALineC0 = PathA0(1);
            HWARange = PathRange(1);
            
            HWALeLineValid = PathValid(1);
            HWALeLineC3 = PathA3(1);
            HWALeLineC2 = PathA2(1);
            HWALeLineC1 = PathA1(1);
            HWALeLineC0 = PathA0(1);
            HWALeRange = PathRange(1);
            
            HWARiLineValid = PathValid(2);
            HWARiLineC3 = PathA3(2);
            HWARiLineC2 = PathA2(2);
            HWARiLineC1 = PathA1(2);
            HWARiLineC0 = PathA0(2);
            HWARiRange = PathRange(2);
        elseif MoveID==0
            
            HWALineValid = PathValid(2);
            HWALineC3 = PathA3(2);
            HWALineC2 = PathA2(2);
            HWALineC1 = PathA1(2);
            HWALineC0 = PathA0(2);
            HWARange = PathRange(2);
            
            if PathLaneAvail(1)&&(TJA_Line_State==1)&&(PathA0(1)<4.5)
                HWALeLineValid = PathValid(1);
                HWALeLineC3 = PathA3(1);
                HWALeLineC2 = PathA2(1);
                HWALeLineC1 = PathA1(1);
                HWALeLineC0 = PathA0(1);
                HWALeRange = PathRange(1);
            end
            
            if PathLaneAvail(3)&&(TJA_Line_State==1)&&(PathA0(3)>-4.5)
                HWARiLineValid = PathValid(3);
                HWARiLineC3 = PathA3(3);
                HWARiLineC2 = PathA2(3);
                HWARiLineC1 = PathA1(3);
                HWARiLineC0 = PathA0(3);
                HWARiRange = PathRange(3);
            end
        end
    end
end
if HWASts==6
    if HWAStsK1~=6
        MoveID = MoveID + int8(1);
    end
    if LeftOffset_b
        MoveID = MoveID + int8(1);
    end
    if RightOffset_b
        MoveID = MoveID - int8(1);
    end

    if (MoveID>=2)||(MoveID<=-1)
        Error = true;
    end
    if Error==false
        if MoveID==1
            HWALineValid = PathValid(3);
            HWALineC3 = PathA3(3);
            HWALineC2 = PathA2(3);
            HWALineC1 = PathA1(3);
            HWALineC0 = PathA0(3);
            HWARange = PathRange(3);
            
            HWALeLineValid = PathValid(2);
            HWALeLineC3 = PathA3(2);
            HWALeLineC2 = PathA2(2);
            HWALeLineC1 = PathA1(2);
            HWALeLineC0 = PathA0(2);
            HWALeRange = PathRange(2);
            
            HWARiLineValid = PathValid(3);
            HWARiLineC3 = PathA3(3);
            HWARiLineC2 = PathA2(3);
            HWARiLineC1 = PathA1(3);
            HWARiLineC0 = PathA0(3);
            HWARiRange = PathRange(3);
            
        elseif MoveID==0
            
            HWALineValid = PathValid(2);
            HWALineC3 = PathA3(2);
            HWALineC2 = PathA2(2);
            HWALineC1 = PathA1(2);
            HWALineC0 = PathA0(2);
            HWARange = PathRange(2);
            
            if PathLaneAvail(1)&&(TJA_Line_State==1)&&(PathA0(1)<4.5)
                HWALeLineValid = PathValid(1);
                HWALeLineC3 = PathA3(1);
                HWALeLineC2 = PathA2(1);
                HWALeLineC1 = PathA1(1);
                HWALeLineC0 = PathA0(1);
                HWALeRange = PathRange(1);
            end
            
            if PathLaneAvail(3)&&(TJA_Line_State==1)&&(PathA0(3)>-4.5)
                HWARiLineValid = PathValid(3);
                HWARiLineC3 = PathA3(3);
                HWARiLineC2 = PathA2(3);
                HWARiLineC1 = PathA1(3);
                HWARiLineC0 = PathA0(3);
                HWARiRange = PathRange(3);
            end
        end
    end
end


%% Double Line Lost
t_Dist = max(single(15),vRef*1.8);
x = [0.05*t_Dist;0.3*t_Dist;0.6*t_Dist;t_Dist];
t_dx = x-dDeltaX;
Y_Tar = HWALineC3*x.^3 + HWALineC2*x.^2 + HWALineC1*x + HWALineC0;
dy_Tar = Y_Tar-dDeltaY;
TmpX = t_dx*CosOfPsi+dy_Tar*SinOfPsi;
TmpY = -t_dx*SinOfPsi+dy_Tar*CosOfPsi;
[~,~,HeadAng_Error,preDyDiff] = pl(TmpX,TmpY);
HeadAngDiff = atan(HeadAng_Error)*57.3;
% xOffset = single(2.1);
%
% t_dyDiff = HWALineA3*xOffset^3 + HWALineA2*xOffset^2 + HWALineA1*xOffset + HWALineA0;
% t_A1 = 3*HWALineA3*xOffset^2 + 2*HWALineA2*xOffset + HWALineA1;
% dyDiff = t_dyDiff/sqrt(single(1) + t_A1^2);

== matlab function PvtSubSys_LSM/Subsystem/TargetLineCalc_20ms/TargetLineCalc/LREWidthCalc ==
  data: LRELineConf input uint8 size=2; a1 input single size=2; a0 input single size=2; LRELineUpdate input boolean size=1; LREWidthK1 input single size=1; LREWidth output single size=1
function LREWidth  = VisRoadWidth(LRELineConf,a1,a0,LRELineUpdate,LREWidthK1)

LREWidth = LREWidthK1;
Update = false;
temp = single(0);

if LRELineUpdate
    if (LRELineConf(1)>0)&&(LRELineConf(2)>0)
        if abs(57.3*(atan(a1(1)) - atan(a1(2))))<3
            temp = (a0(1) - a0(2))/sqrt(a1(2)^2 + single(1));
            Update = true;
        end
    end
    if Update
        LREWidth = 0.1*(temp - LREWidthK1) + LREWidthK1;
    end
end

== matlab function PvtSubSys_LSM/Subsystem/TargetLineCalc_20ms/TargetLineCalc/MATLAB Function1 ==
  data: HWASts input uint8 size=1; HWALeLineValid output boolean size=1; RoadWidth input single size=1; LineValid input boolean size=1; LineC3 input single size=1; LineC2 input single size=1; LineC1 input single size=1; LineC0 input single size=1; LineRange input single size=1; LeLineValid input boolean size=1; LeLineC3 input single size=1; LeLineC2 input single size=1; LeLineC1 input single size=1; LeLineC0 input single size=1; LeLineRange input single size=1; RiLineValid input boolean size=1; RiLineC3 input single size=1; RiLineC2 input single size=1; RiLineC1 input single size=1; RiLineC0 input single size=1; RiLineRange input single size=1; HWALeLineC3 output single size=1; HWALeLineC2 output single size=1; HWALeLineC1 output single size=1; HWALeLineC0 output single size=1; HWALeLineRange output single size=1; LeLineVirtual_b output boolean size=1; HWARiLineValid output boolean size=1; HWARiLineC3 output single size=1; HWARiLineC2 output single size=1; HWARiLineC1 output single size=1; HWARiLineC0 output single size=1; HWARiLineRange output single size=1; RiLineVirtual_b output boolean size=1
function [HWALeLineValid,HWALeLineC3,HWALeLineC2,HWALeLineC1,HWALeLineC0,HWALeLineRange,LeLineVirtual_b,...
    HWARiLineValid,HWARiLineC3,HWARiLineC2,HWARiLineC1,HWARiLineC0,HWARiLineRange,RiLineVirtual_b]...
    = LineAddCalc(HWASts,RoadWidth,LineValid,LineC3,LineC2,LineC1,LineC0,LineRange,...
    LeLineValid,LeLineC3,LeLineC2,LeLineC1,LeLineC0,LeLineRange,...
    RiLineValid,RiLineC3,RiLineC2,RiLineC1,RiLineC0,RiLineRange)

if LeLineValid==true||HWASts~=3
    HWALeLineValid = LeLineValid;
    HWALeLineC3 = LeLineC3;
    HWALeLineC2 = LeLineC2;
    HWALeLineC1 = LeLineC1;
    HWALeLineC0 = LeLineC0;
    HWALeLineRange = LeLineRange;
    LeLineVirtual_b = false;
else
    HWALeLineValid = false;
    HWALeLineC3 = LineC3;
    HWALeLineC2 = LineC2;
    HWALeLineC1 = LineC1;
    HWALeLineC0 = LineC0 + RoadWidth;
    HWALeLineRange = LineRange;
    LeLineVirtual_b = true;
end

if RiLineValid==true||HWASts~=3
    HWARiLineValid = RiLineValid;
    HWARiLineC3 = RiLineC3;
    HWARiLineC2 = RiLineC2;
    HWARiLineC1 = RiLineC1;
    HWARiLineC0 = RiLineC0;
    HWARiLineRange = RiLineRange;
    RiLineVirtual_b = false;
else
    HWARiLineValid = false;
    HWARiLineC3 = LineC3;
    HWARiLineC2 = LineC2;
    HWARiLineC1 = LineC1;
    HWARiLineC0 = LineC0 - RoadWidth;
    HWARiLineRange = LineRange;
    RiLineVirtual_b = true;
end
